simulink model "VSCHVDCunitblackstart"  (R2025b)
settings: Solver=VariableStepAuto  StartTime=0  StopTime=25  FixedStep=5e-5  RelTol=1e-3
PreLoadFcn:
  | HVDCParameters;
  | BlackStartMMCParameters;
undefined symbols (not defined in the file): DiscIntNeverNeededParam, FRated, frt, gGFM, grid, Lbase, Lr, Lt, lvrt, mGFM, mpptOmega, mpptWindSpeed, Nm, pmsm, PRated, Rc, rpir, Rr, Rt, time, Tpir, Ts, Vbase, Vdcs0, VRated, Vt2, windController, windTurbine, Zbase
libraries: fl_lib x47, ee_lib x41, nesl_utility x33, eeGeneralControl x13, eeTransforms x12, slpidlib x8, eeSinusoidalMeasurementV2 x4, simulink x2, eeSinusoidalMeasurement x1, eeStairGenerator x1
(part 5 of 5)

== system VSCHVDCunitblackstart/Control/Sending-end and receiving-end control/Onshore Control/Control/Active and reactive power control ==
  Vd : Inport
  Vdmea : Inport  Port=2
  Vqref : Inport  Port=3
  Vqmea : Inport  Port=4
  P PI : slpidlib/PID Controller  Controller=PI  Form=Parallel  TimeDomain=Discrete-time  UseExternalTs=off  SampleTime=Tsc  IntegratorMethod=Forward Euler  FilterMethod=Forward Euler  ControllerParametersSource=internal  P=1  I=SEnd_P_PI(2)  UseKiTs=off  D=0  UseExternalDerivativeSource=off  N=100  UseFilter=on  TunerSelectOption=Transfer Function Based (PID Tuner App)  InitialConditionSource=internal  InitialConditionForIntegrator=0  InitialConditionForFilter=0  DifferentiatorICPrevScaledInput=0  ExternalReset=none  TrackingMode=off  Kt=1  LimitOutput=off  SatLimitsSource=internal  UpperSaturationLimit=1.1  LowerSaturationLimit=0  LinearizeAsGain=on  AntiWindupMode=back-calculation  Kb=1000  LimitIntegrator=off  UpperIntegratorSaturationLimit=inf  LowerIntegratorSaturationLimit=-inf  POutMin=[]  POutMax=[]  IOutMin=[]  IOutMax=[]  DOutMin=[]  DOutMax=[]  NOutMin=[]  NOutMax=[]  SumOutMin=[]  SumOutMax=[]  SaturationOutMin=[]  SaturationOutMax=[]  PParamMin=[]  PParamMax=[]  IParamMin=[]  IParamMax=[]  DParamMin=[]  DParamMax=[]  NParamMin=[]  NParamMax=[]  KbParamMin=[]  KbParamMax=[]  KtParamMin=[]  KtParamMax=[]  KbOutMin=[]  KbOutMax=[]  KtOutMin=[]  KtOutMax=[]  IntegratorOutMin=[]  IntegratorOutMax=[]  FilterOutMin=[]  FilterOutMax=[]  SumI1OutMin=[]  SumI1OutMax=[]  SumI2OutMin=[]  SumI2OutMax=[]  SumI3OutMin=[]  SumI3OutMax=[]  SumI4OutMin=[]  SumI4OutMax=[]  SumDOutMin=[]  SumDOutMax=[]  DifferentiatorOutMin=[]  DifferentiatorOutMax=[]  FilterDiffOutCoefMin=[]  FilterDiffOutCoefMax=[]  ReciprocalOutMin=[]  ReciprocalOutMax=[]  SumDenOutMin=[]  SumDenOutMax=[]  SumNumOutMin=[]  SumNumOutMax=[]  DivideOutMin=[]  DivideOutMax=[]  UdiffTsProdOutMin=[]  UdiffTsProdOutMax=[]  NTsProdOutMin=[]  NTsProdOutMax=[]  UintegralTsProdOutMin=[]  UintegralTsProdOutMax=[]  UngainTsProdOutMin=[]  UngainTsProdOutMax=[]  ClampingZeroOutDataTypeStr=Inherit: Inherit via back propagation  ClampingZeroOutMin=[]  ClampingZeroOutMax=[]  FilterDenConstantOutDataTypeStr=Inherit: Inherit via back propagation  FilterDenConstantOutMin=[]  FilterDenConstantOutMax=[]  PCopyOutDataTypeStr=Inherit: Inherit via back propagation  PCopyOutMin=[]  PCopyOutMax=[]  NCopyOutDataTypeStr=Inherit: Inherit via back propagation  NCopyOutMin=[]  NCopyOutMax=[]  IntegratorContinuousStateAttributes=''  IntegratorStateMustResolveToSignalObject=off  IntegratorRTWStateStorageClass=Auto  FilterContinuousStateAttributes=''  FilterStateMustResolveToSignalObject=off  FilterRTWStateStorageClass=Auto  ParallelPVariant=InternalParameters  IdealPVariant=Disabled  IVariant=InternalParameters  DVariant=Disabled  IntegratorVariant=Discrete  SatVariant=Disabled  AWVariant=Passthrough  PCopyVariant=Disabled  TRVariant=Disabled  FdbkBlocksVariant=Forward  IdealPFdbkVariant=Disabled  SatFdbkVariant=Disabled  DerivativeFilterVariant=Disabled  NVariant=Disabled  NCopyVariant=Disabled_SignalSpec  FilterICVariant=Disabled  IntegratorICVariant=InternalICs  ExternalResetVariant=Disabled  TRSumVariant=Passthrough  SumFdbkVariant=Disabled  SumVariant=Sum_PI  TsampFilterVariant=InternalTs  TsampNgainVariant=Passthrough  TsampIntegralVariant=Disabled_SignalSpec  ExternalSaturationOutDataTypeStr=Inherit: Same as second input  DerivativeSourceVariant=Disabled  PreIntVariant=InternalPreInt
  P PI1 : slpidlib/PID Controller  Controller=PI  Form=Parallel  TimeDomain=Discrete-time  UseExternalTs=off  SampleTime=Tsc  IntegratorMethod=Forward Euler  FilterMethod=Forward Euler  ControllerParametersSource=internal  P=1  I=SEnd_P_PI(2)  UseKiTs=off  D=0  UseExternalDerivativeSource=off  N=100  UseFilter=on  TunerSelectOption=Transfer Function Based (PID Tuner App)  InitialConditionSource=internal  InitialConditionForIntegrator=0  InitialConditionForFilter=0  DifferentiatorICPrevScaledInput=0  ExternalReset=none  TrackingMode=off  Kt=1  LimitOutput=off  SatLimitsSource=internal  UpperSaturationLimit=1.5  LowerSaturationLimit=-.0  LinearizeAsGain=on  AntiWindupMode=back-calculation  Kb=1000  LimitIntegrator=off  UpperIntegratorSaturationLimit=inf  LowerIntegratorSaturationLimit=-inf  POutMin=[]  POutMax=[]  IOutMin=[]  IOutMax=[]  DOutMin=[]  DOutMax=[]  NOutMin=[]  NOutMax=[]  SumOutMin=[]  SumOutMax=[]  SaturationOutMin=[]  SaturationOutMax=[]  PParamMin=[]  PParamMax=[]  IParamMin=[]  IParamMax=[]  DParamMin=[]  DParamMax=[]  NParamMin=[]  NParamMax=[]  KbParamMin=[]  KbParamMax=[]  KtParamMin=[]  KtParamMax=[]  KbOutMin=[]  KbOutMax=[]  KtOutMin=[]  KtOutMax=[]  IntegratorOutMin=[]  IntegratorOutMax=[]  FilterOutMin=[]  FilterOutMax=[]  SumI1OutMin=[]  SumI1OutMax=[]  SumI2OutMin=[]  SumI2OutMax=[]  SumI3OutMin=[]  SumI3OutMax=[]  SumI4OutMin=[]  SumI4OutMax=[]  SumDOutMin=[]  SumDOutMax=[]  DifferentiatorOutMin=[]  DifferentiatorOutMax=[]  FilterDiffOutCoefMin=[]  FilterDiffOutCoefMax=[]  ReciprocalOutMin=[]  ReciprocalOutMax=[]  SumDenOutMin=[]  SumDenOutMax=[]  SumNumOutMin=[]  SumNumOutMax=[]  DivideOutMin=[]  DivideOutMax=[]  UdiffTsProdOutMin=[]  UdiffTsProdOutMax=[]  NTsProdOutMin=[]  NTsProdOutMax=[]  UintegralTsProdOutMin=[]  UintegralTsProdOutMax=[]  UngainTsProdOutMin=[]  UngainTsProdOutMax=[]  ClampingZeroOutDataTypeStr=Inherit: Inherit via back propagation  ClampingZeroOutMin=[]  ClampingZeroOutMax=[]  FilterDenConstantOutDataTypeStr=Inherit: Inherit via back propagation  FilterDenConstantOutMin=[]  FilterDenConstantOutMax=[]  PCopyOutDataTypeStr=Inherit: Inherit via back propagation  PCopyOutMin=[]  PCopyOutMax=[]  NCopyOutDataTypeStr=Inherit: Inherit via back propagation  NCopyOutMin=[]  NCopyOutMax=[]  IntegratorContinuousStateAttributes=''  IntegratorStateMustResolveToSignalObject=off  IntegratorRTWStateStorageClass=Auto  FilterContinuousStateAttributes=''  FilterStateMustResolveToSignalObject=off  FilterRTWStateStorageClass=Auto  ParallelPVariant=InternalParameters  IdealPVariant=Disabled  IVariant=InternalParameters  DVariant=Disabled  IntegratorVariant=Discrete  SatVariant=Disabled  AWVariant=Passthrough  PCopyVariant=Disabled  TRVariant=Disabled  FdbkBlocksVariant=Forward  IdealPFdbkVariant=Disabled  SatFdbkVariant=Disabled  DerivativeFilterVariant=Disabled  NVariant=Disabled  NCopyVariant=Disabled_SignalSpec  FilterICVariant=Disabled  IntegratorICVariant=InternalICs  ExternalResetVariant=Disabled  TRSumVariant=Passthrough  SumFdbkVariant=Disabled  SumVariant=Sum_PI  TsampFilterVariant=InternalTs  TsampNgainVariant=Passthrough  TsampIntegralVariant=Disabled_SignalSpec  ExternalSaturationOutDataTypeStr=Inherit: Same as second input  DerivativeSourceVariant=Disabled  PreIntVariant=InternalPreInt
  Sum5 : Sum  Inputs=|+-
  Sum6 : Sum  Inputs=|+-
  idRef : Outport
  iqRef : Outport  Port=2
  wires:
  P PI1/1 -> iqRef/1
  P PI/1 -> idRef/1
  Sum5/1 -> P PI/1
  Sum6/1 -> P PI1/1
  Vqref/1 -> Sum6/1
  Vqmea/1 -> Sum6/2
  Vd/1 -> Sum5/1
  Vdmea/1 -> Sum5/2

== system VSCHVDCunitblackstart/Control/Sending-end and receiving-end control/Onshore Control/Control/PWM generator ==
  Vref : Inport
  Gain4 : Gain  Gain=-1
  Mux2 : Mux  Inputs=2
  Selector : Selector  InputPortWidth=6  IndexOptions=Index vector (dialog)  Indices=[1 4 2 5 3 6]  OutputSizes=1
  S : Outport
  wires:
  Mux2/1 -> Selector/1
  Vref/1 -> Mux2/2, Gain4/1
  Gain4/1 -> Mux2/1
  Selector/1 -> S/1

== system VSCHVDCunitblackstart/Control/Sending-end and receiving-end control/Onshore Control/Measurements/PQ Calculation ==
  Vd : Inport
  Id : Inport  Port=2
  Iq : Inport  Port=3
  Gain : Gain  Gain=-1
  Product : Product
  Product4 : Product
  P : Outport
  Q : Outport  Port=2
  wires:
  Vd/1 -> Product4/1, Product/1
  Product/1 -> P/1
  Id/1 -> Product/2
  Iq/1 -> Product4/2
  Product4/1 -> Gain/1
  Gain/1 -> Q/1

== system VSCHVDCunitblackstart/Control/Sending-end and receiving-end control/Onshore Control/Measurements/Subsystem ==
  In : Inport
  Gain2 : Gain  Gain=2
  Sum2 : Sum  Inputs=+-  InputSameDT=on  SaturateOnIntegerOverflow=on  OutDataTypeStr=Inherit: Same as first input
  Unit Delay4 : UnitDelay  InitialCondition=Iabcgs0  SampleTime=Ts  HasFrameUpgradeWarning=on
  Out : Outport
  wires:
  Unit Delay4/1 -> Sum2/2
  Sum2/1 -> Out/1
  Gain2/1 -> Sum2/1
  In/1 -> Gain2/1, Unit Delay4/1

== system VSCHVDCunitblackstart/Control/Sending-end and receiving-end control/Onshore Control/Measurements/Subsystem1 ==
  In : Inport
  Gain2 : Gain  Gain=2
  Sum2 : Sum  Inputs=+-  InputSameDT=on  SaturateOnIntegerOverflow=on  OutDataTypeStr=Inherit: Same as first input
  Unit Delay4 : UnitDelay  InitialCondition=Vabcgs0  SampleTime=Ts  HasFrameUpgradeWarning=on
  Out : Outport
  wires:
  In/1 -> Unit Delay4/1, Gain2/1
  Gain2/1 -> Sum2/1
  Sum2/1 -> Out/1
  Unit Delay4/1 -> Sum2/2

== system VSCHVDCunitblackstart/Wind Farm/Wind Farm/Voltage VAR Control & LVRT, FRT/Frequency RideThrough/Avoid Operation ==
  f_in : Inport
  Constant : Constant  Value=grid.frequency  SampleTime=Ts
  Step : Step  Time=0.5  SampleTime=Ts
  Switch : Switch  Criteria=u2 > Threshold  SaturateOnIntegerOverflow=off  InputSameDT=off
  f : Outport
  wires:
  f_in/1 -> Switch/1
  Constant/1 -> Switch/3
  Step/1 -> Switch/2
  Switch/1 -> f/1

== system VSCHVDCunitblackstart/Wind Farm/Wind Farm1/Voltage VAR Control & LVRT, FRT/Frequency RideThrough/Avoid Operation ==
  f_in : Inport
  Constant : Constant  Value=grid.frequency  SampleTime=Ts
  Step : Step  Time=0.5  SampleTime=Ts
  Switch : Switch  Criteria=u2 > Threshold  SaturateOnIntegerOverflow=off  InputSameDT=off
  f : Outport
  wires:
  f_in/1 -> Switch/1
  Constant/1 -> Switch/3
  Step/1 -> Switch/2
  Switch/1 -> f/1
